simulink model "H16"  (Simulink 7.3)
settings: Solver=ode45  StartTime=0.0  StopTime=2  RelTol=1e-3
undefined symbols (not defined in the file or in its folder): DiscIntNeverNeededParam
libraries: simulink x13
settings Model: Creator=Sainquake  LastModifiedBy=Sainquake

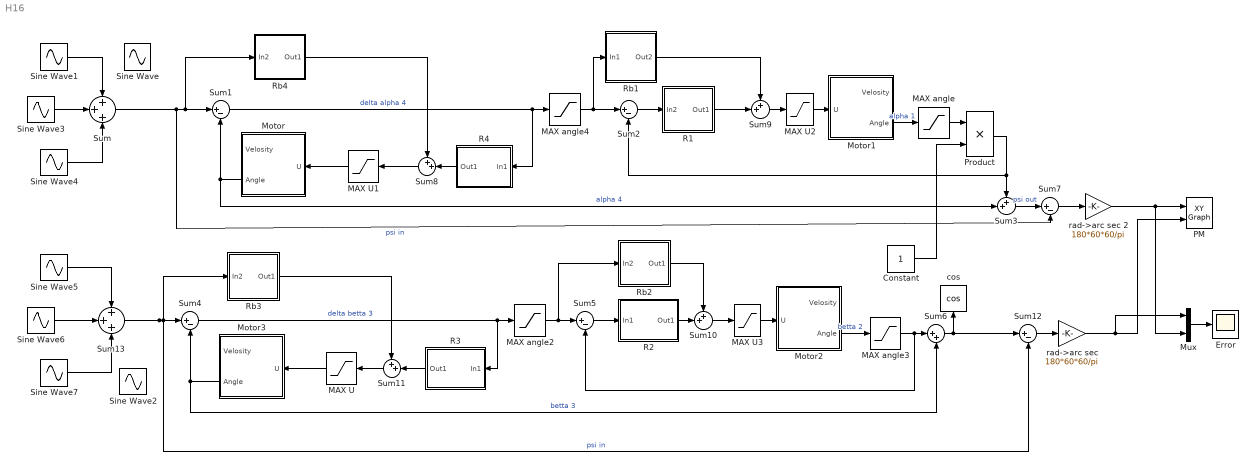
== system H16 ==
  Constant : Constant  OutDataType=fixdt(1, 16)  OutScaling=2^0
  Error : Scope
      settings: YMin=-50  YMax=250  SaveName=ScopeData2  MaxDataPoints=500000
  MAX U : Saturate  UpperLimit=42  LowerLimit=-42
  MAX U1 : Saturate  UpperLimit=42  LowerLimit=-42
  MAX U2 : Saturate  UpperLimit=12  LowerLimit=-12
  MAX U3 : Saturate  UpperLimit=12  LowerLimit=-12
  MAX angle : Saturate  UpperLimit=8/180*3.14  LowerLimit=-8/180*3.14
  MAX angle2 : Saturate  UpperLimit=4/180*3.14  LowerLimit=-4/180*3.14
  MAX angle3 : Saturate  UpperLimit=4/180*3.14  LowerLimit=-4/180*3.14
  MAX angle4 : Saturate  UpperLimit=8/180*3.14  LowerLimit=-8/180*3.14
  Motor : Subsystem  TreatAsAtomicUnit=on
  Motor1 : Subsystem  TreatAsAtomicUnit=on
  Motor2 : Subsystem  TreatAsAtomicUnit=on
  Motor3 : Subsystem  TreatAsAtomicUnit=on
  Mux : Mux  Inputs=2
  PM : simulink/Sinks/XY Graph  SystemSampleTime=-1  xmin=-3*1280  xmax=3*1280  ymin=-3*960  ymax=3*960  st=-1
  Product : Product  OutDataType=fixdt(1, 16)  OutScaling=2^0  RndMeth=Zero
  R1 : Subsystem
  R2 : Subsystem
  R3 : Subsystem
  R4 : Subsystem
  Rb1 : Subsystem
  Rb2 : Subsystem
  Rb3 : Subsystem
  Rb4 : Subsystem
  Sine Wave{,1..2,5} (4 alike) : Sin  Amplitude=1  Bias=0  Frequency=1  Phase=0  Samples=10  SampleTime=0  Offset=0
  Sine Wave3 : Sin  Amplitude=1/10000  Bias=0  Frequency=2*pi*14  Phase=0  Samples=10  SampleTime=0  Offset=0
  Sine Wave4 : Sin  Amplitude=1/400  Bias=0  Frequency=2*pi*4  Phase=0  Samples=10  SampleTime=0  Offset=0
  Sine Wave6 : Sin  Amplitude=1/10000  Bias=0  Frequency=2*pi*14  Phase=0  Samples=10  SampleTime=0  Offset=0
  Sine Wave7 : Sin  Amplitude=1/400  Bias=0  Frequency=2*pi*4  Phase=0  Samples=10  SampleTime=0  Offset=0
  Sum : Sum  Inputs=+++  OutDataType=fixdt(1, 16)  OutScaling=2^0
  Sum{1..2,4..5,7,12} (6 alike) : Sum  Inputs=|+-  OutDataType=fixdt(1, 16)  OutScaling=2^0
  Sum{3,8..11} (5 alike) : Sum  Inputs=++|  OutDataType=fixdt(1, 16)  OutScaling=2^0
  Sum13 : Sum  Inputs=+++  OutDataType=fixdt(1, 16)  OutScaling=2^0
  Sum6 : Sum  Inputs=|++  OutDataType=fixdt(1, 16)  OutScaling=2^0
  cos : Trigonometry  Operator=cos
  rad->arc sec : Gain  Gain=180*60*60/pi  ParameterDataType=fixdt(1, 16)  ParameterScaling=2^0  OutDataType=fixdt(1, 16)  OutScaling=2^0
  rad->arc sec 2 : Gain  Gain=180*60*60/pi  ParameterDataType=fixdt(1, 16)  ParameterScaling=2^0  OutDataType=fixdt(1, 16)  OutScaling=2^0
  wires:
  R4/1(Out1) -> Sum8/2
  Motor1/2(Angle) -> MAX angle/1  "alpha 1"
  Sum2/1 -> R1/1(In2)
  Product/1 -> Sum3/1, Sum2/2
  Sum3/1 -> Sum7/1  "psi out"
  Motor/2(Angle) -> Sum1/2, Sum3/2  "alpha 4"
  R3/1(Out1) -> Sum11/2
  Sum4/1 -> R3/1(In1), MAX angle2/1  "delta betta 3"
  Sum13/1 -> Sum4/1, Rb3/1(In2), Sum12/2  "psi in"
  R2/1(Out1) -> Sum10/2
  Motor2/2(Angle) -> MAX angle3/1  "betta 2"
  Sum5/1 -> R2/1(In1)
  Motor3/2(Angle) -> Sum4/2, Sum6/2  "betta 3"
  Sum6/1 -> cos/1, Sum12/1
  Sum/1 -> Sum1/1, Rb4/1(In2), Sum7/2  "psi in"
  Rb1/1(Out2) -> Sum9/1
  Rb4/1(Out1) -> Sum8/1
  R1/1(Out1) -> Sum9/2
  Sum9/1 -> MAX U2/1
  Rb3/1(Out1) -> Sum11/1
  Sum11/1 -> MAX U/1
  Sum10/1 -> MAX U3/1
  Rb2/1(Out1) -> Sum10/1
  Sum7/1 -> rad->arc sec 2/1
  rad->arc sec 2/1 -> PM/1, Mux/2
  Sum1/1 -> R4/1(In1), MAX angle4/1  "delta alpha 4"
  rad->arc sec/1 -> Mux/1, PM/2
  Sum12/1 -> rad->arc sec/1
  Mux/1 -> Error/1
  MAX angle4/1 -> Sum2/1, Rb1/1(In1)
  MAX angle2/1 -> Sum5/1, Rb2/1(In2)
  MAX U2/1 -> Motor1/1(U)
  MAX U3/1 -> Motor2/1(U)
  MAX angle/1 -> Product/1
  MAX angle3/1 -> Sum5/2, Sum6/1
  Sum8/1 -> MAX U1/1
  MAX U/1 -> Motor3/1(U)
  MAX U1/1 -> Motor/1(U)
  Sine Wave3/1 -> Sum/2
  Sine Wave1/1 -> Sum/1
  Sine Wave6/1 -> Sum13/2
  Sine Wave7/1 -> Sum13/3
  Sine Wave4/1 -> Sum/3
  Sine Wave5/1 -> Sum13/1
  Constant/1 -> Product/2

== system H16/Motor ==
  U : Inport  OutDataType=fixdt(1, 16)  OutScaling=2^0
  Ang : Integrator
  Transfer Fcn3 : TransferFcn  Numerator=[3.87]  Denominator=[16.713 1]
  Velosity : Outport  OutDataType=fixdt(1, 16)  OutScaling=2^0
  Angle : Outport  Port=2  OutDataType=fixdt(1, 16)  OutScaling=2^0
  wires:
  Ang/1 -> Angle/1
  U/1 -> Transfer Fcn3/1
  Transfer Fcn3/1 -> Ang/1, Velosity/1

== system H16/Motor1 ==
  U : Inport  OutDataType=fixdt(1, 16)  OutScaling=2^0
  Ang : Integrator
  Transfer Fcn3 : TransferFcn  Numerator=[8.37]  Denominator=[0.0002343 1]
  Velosity : Outport  OutDataType=fixdt(1, 16)  OutScaling=2^0
  Angle : Outport  Port=2  OutDataType=fixdt(1, 16)  OutScaling=2^0
  wires:
  Ang/1 -> Angle/1
  U/1 -> Transfer Fcn3/1
  Transfer Fcn3/1 -> Ang/1, Velosity/1

== system H16/Motor2 ==
  U : Inport  OutDataType=fixdt(1, 16)  OutScaling=2^0
  Ang : Integrator
  Transfer Fcn3 : TransferFcn  Numerator=[8.37]  Denominator=[0.015 1]
  Velosity : Outport  OutDataType=fixdt(1, 16)  OutScaling=2^0
  Angle : Outport  Port=2  OutDataType=fixdt(1, 16)  OutScaling=2^0
  wires:
  Ang/1 -> Angle/1
  U/1 -> Transfer Fcn3/1
  Transfer Fcn3/1 -> Ang/1, Velosity/1

== system H16/Motor3 ==
  U : Inport  OutDataType=fixdt(1, 16)  OutScaling=2^0
  Ang : Integrator
  Transfer Fcn3 : TransferFcn  Numerator=[3.87]  Denominator=[2.662 1]
  Velosity : Outport  OutDataType=fixdt(1, 16)  OutScaling=2^0
  Angle : Outport  Port=2  OutDataType=fixdt(1, 16)  OutScaling=2^0
  wires:
  Ang/1 -> Angle/1
  U/1 -> Transfer Fcn3/1
  Transfer Fcn3/1 -> Ang/1, Velosity/1

== system H16/R1 ==
  In2 : Inport  OutDataType=fixdt(1, 16)  OutScaling=2^0
  Constan : Constant  Value=1935.48  OutDataType=fixdt(1, 16)  OutScaling=2^0
  Constan1 : Constant  Value=0  OutDataType=fixdt(1, 16)  OutScaling=2^0
  Constan2 : Constant  Value=0.453  OutDataType=fixdt(1, 16)  OutScaling=2^0
  PID : Subsystem
  Out1 : Outport  OutDataType=fixdt(1, 16)  OutScaling=2^0
  wires:
  Constan/1 -> PID/2(p)
  Constan1/1 -> PID/3(i)
  Constan2/1 -> PID/4(d)
  In2/1 -> PID/1(In1)
  PID/1(Out1) -> Out1/1

== system H16/R2 ==
  In1 : Inport  OutDataType=fixdt(1, 16)  OutScaling=2^0
  Constan : Constant  Value=645.161*5  OutDataType=fixdt(1, 16)  OutScaling=2^0
  Constan1 : Constant  Value=0  OutDataType=fixdt(1, 16)  OutScaling=2^0
  Constan2 : Constant  Value=645.161*5*0.015/10  OutDataType=fixdt(1, 16)  OutScaling=2^0
  PID : Subsystem
  Out1 : Outport  OutDataType=fixdt(1, 16)  OutScaling=2^0
  wires:
  Constan/1 -> PID/2(p)
  Constan1/1 -> PID/3(i)
  Constan2/1 -> PID/4(d)
  In1/1 -> PID/1(In1)
  PID/1(Out1) -> Out1/1

== system H16/R3 ==
  In1 : Inport  OutDataType=fixdt(1, 16)  OutScaling=2^0
  Constan : Constant  Value=755/10  OutDataType=fixdt(1, 16)  OutScaling=2^0
  Constan1 : Constant  Value=0  OutDataType=fixdt(1, 16)  OutScaling=2^0
  Constan2 : Constant  Value=2.662*775/10  OutDataType=fixdt(1, 16)  OutScaling=2^0
  PID : Subsystem
  Out1 : Outport  OutDataType=fixdt(1, 16)  OutScaling=2^0
  wires:
  Constan/1 -> PID/2(p)
  Constan1/1 -> PID/3(i)
  Constan2/1 -> PID/4(d)
  In1/1 -> PID/1(In1)
  PID/1(Out1) -> Out1/1

== system H16/R4 ==
  In1 : Inport  OutDataType=fixdt(1, 16)  OutScaling=2^0
  Constan : Constant  Value=755/10  OutDataType=fixdt(1, 16)  OutScaling=2^0
  Constan1 : Constant  Value=0  OutDataType=fixdt(1, 16)  OutScaling=2^0
  Constan2 : Constant  Value=12952.57/10  OutDataType=fixdt(1, 16)  OutScaling=2^0
  PID : Subsystem
  Out1 : Outport  OutDataType=fixdt(1, 16)  OutScaling=2^0
  wires:
  In1/1 -> PID/1(In1)
  Constan/1 -> PID/2(p)
  Constan1/1 -> PID/3(i)
  Constan2/1 -> PID/4(d)
  PID/1(Out1) -> Out1/1

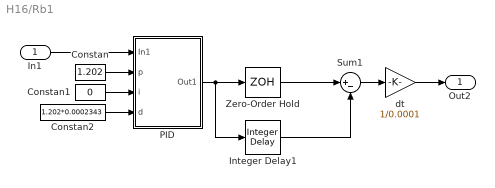
== system H16/Rb1 ==
  In1 : Inport  OutDataType=fixdt(1, 16)  OutScaling=2^0
  Constan : Constant  Value=1.202  OutDataType=fixdt(1, 16)  OutScaling=2^0
  Constan1 : Constant  Value=0  OutDataType=fixdt(1, 16)  OutScaling=2^0
  Constan2 : Constant  Value=1.202*0.0002343  OutDataType=fixdt(1, 16)  OutScaling=2^0
  Integer Delay1 : simulink/Discrete/Integer Delay  vinit=0  samptime=0.0001  NumDelays=1
  PID : Subsystem
  Sum1 : Sum  Inputs=|+-  OutDataType=fixdt(1, 16)  OutScaling=2^0
  Zero-Order Hold : ZeroOrderHold  SampleTime=0.0001
  dt : Gain  Gain=1/0.0001  ParameterDataType=fixdt(1, 16)  ParameterScaling=2^0  OutDataType=fixdt(1, 16)  OutScaling=2^0
  Out2 : Outport  OutDataType=fixdt(1, 16)  OutScaling=2^0
  wires:
  Constan/1 -> PID/2(p)
  Constan1/1 -> PID/3(i)
  Constan2/1 -> PID/4(d)
  Zero-Order Hold/1 -> Sum1/1
  Sum1/1 -> dt/1
  Integer Delay1/1 -> Sum1/2
  PID/1(Out1) -> Integer Delay1/1, Zero-Order Hold/1
  In1/1 -> PID/1(In1)
  dt/1 -> Out2/1

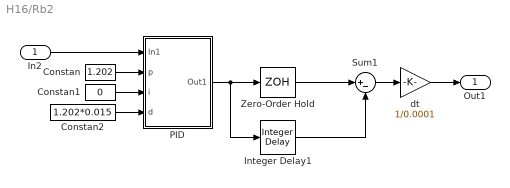
== system H16/Rb2 ==
  In2 : Inport  OutDataType=fixdt(1, 16)  OutScaling=2^0
  Constan : Constant  Value=1.202  OutDataType=fixdt(1, 16)  OutScaling=2^0
  Constan1 : Constant  Value=0  OutDataType=fixdt(1, 16)  OutScaling=2^0
  Constan2 : Constant  Value=1.202*0.015  OutDataType=fixdt(1, 16)  OutScaling=2^0
  Integer Delay1 : simulink/Discrete/Integer Delay  vinit=0  samptime=0.0001  NumDelays=1
  PID : Subsystem
  Sum1 : Sum  Inputs=|+-  OutDataType=fixdt(1, 16)  OutScaling=2^0
  Zero-Order Hold : ZeroOrderHold  SampleTime=0.0001
  dt : Gain  Gain=1/0.0001  ParameterDataType=fixdt(1, 16)  ParameterScaling=2^0  OutDataType=fixdt(1, 16)  OutScaling=2^0
  Out1 : Outport  OutDataType=fixdt(1, 16)  OutScaling=2^0
  wires:
  Constan/1 -> PID/2(p)
  Constan1/1 -> PID/3(i)
  Constan2/1 -> PID/4(d)
  In2/1 -> PID/1(In1)
  Zero-Order Hold/1 -> Sum1/1
  Sum1/1 -> dt/1
  Integer Delay1/1 -> Sum1/2
  PID/1(Out1) -> Integer Delay1/1, Zero-Order Hold/1
  dt/1 -> Out1/1

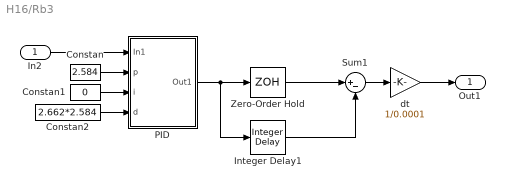
== system H16/Rb3 ==
  In2 : Inport  OutDataType=fixdt(1, 16)  OutScaling=2^0
  Constan : Constant  Value=2.584  OutDataType=fixdt(1, 16)  OutScaling=2^0
  Constan1 : Constant  Value=0  OutDataType=fixdt(1, 16)  OutScaling=2^0
  Constan2 : Constant  Value=2.662*2.584  OutDataType=fixdt(1, 16)  OutScaling=2^0
  Integer Delay1 : simulink/Discrete/Integer Delay  vinit=0  samptime=0.0001  NumDelays=1
  PID : Subsystem
  Sum1 : Sum  Inputs=|+-  OutDataType=fixdt(1, 16)  OutScaling=2^0
  Zero-Order Hold : ZeroOrderHold  SampleTime=0.0001
  dt : Gain  Gain=1/0.0001  ParameterDataType=fixdt(1, 16)  ParameterScaling=2^0  OutDataType=fixdt(1, 16)  OutScaling=2^0
  Out1 : Outport  OutDataType=fixdt(1, 16)  OutScaling=2^0
  wires:
  Constan/1 -> PID/2(p)
  Constan1/1 -> PID/3(i)
  Constan2/1 -> PID/4(d)
  In2/1 -> PID/1(In1)
  Zero-Order Hold/1 -> Sum1/1
  Sum1/1 -> dt/1
  Integer Delay1/1 -> Sum1/2
  PID/1(Out1) -> Integer Delay1/1, Zero-Order Hold/1
  dt/1 -> Out1/1

== system H16/Rb4 ==
  In2 : Inport  OutDataType=fixdt(1, 16)  OutScaling=2^0
  Constan : Constant  Value=2.584  OutDataType=fixdt(1, 16)  OutScaling=2^0
  Constan1 : Constant  Value=0  OutDataType=fixdt(1, 16)  OutScaling=2^0
  Constan2 : Constant  Value=43.1863  OutDataType=fixdt(1, 16)  OutScaling=2^0
  Integer Delay1 : simulink/Discrete/Integer Delay  vinit=0  samptime=0.0001  NumDelays=1
  PID : Subsystem
  Sum1 : Sum  Inputs=|+-  OutDataType=fixdt(1, 16)  OutScaling=2^0
  Zero-Order Hold : ZeroOrderHold  SampleTime=0.0001
  dt : Gain  Gain=1/0.0001  ParameterDataType=fixdt(1, 16)  ParameterScaling=2^0  OutDataType=fixdt(1, 16)  OutScaling=2^0
  Out1 : Outport  OutDataType=fixdt(1, 16)  OutScaling=2^0
  wires:
  Constan/1 -> PID/2(p)
  Constan1/1 -> PID/3(i)
  Constan2/1 -> PID/4(d)
  In2/1 -> PID/1(In1)
  Zero-Order Hold/1 -> Sum1/1
  Sum1/1 -> dt/1
  Integer Delay1/1 -> Sum1/2
  dt/1 -> Out1/1
  PID/1(Out1) -> Zero-Order Hold/1, Integer Delay1/1

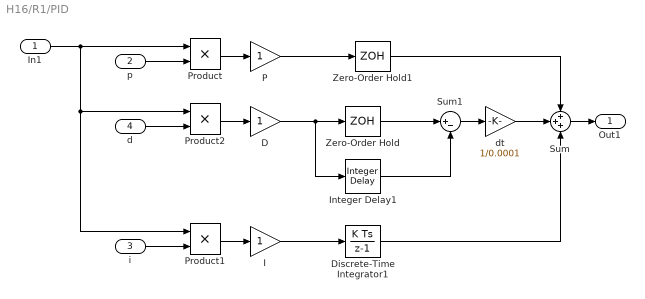
== system H16/R1/PID ==
  In1 : Inport  OutDataType=fixdt(1, 16)  OutScaling=2^0
  p : Inport  Port=2  OutDataType=fixdt(1, 16)  OutScaling=2^0
  i : Inport  Port=3  OutDataType=fixdt(1, 16)  OutScaling=2^0
  d : Inport  Port=4  OutDataType=fixdt(1, 16)  OutScaling=2^0
  D : Gain  ParameterDataType=fixdt(1, 16)  ParameterScaling=2^0  OutDataType=fixdt(1, 16)  OutScaling=2^0
  Discrete-Time Integrator1 : DiscreteIntegrator  SampleTime=0.0001  OutDataType=fixdt(1, 16)  OutScaling=2^0  ICPrevOutput=DiscIntNeverNeededParam  ICPrevScaledInput=DiscIntNeverNeededParam
  I : Gain  ParameterDataType=fixdt(1, 16)  ParameterScaling=2^0  OutDataType=fixdt(1, 16)  OutScaling=2^0
  Integer Delay1 : simulink/Discrete/Integer Delay  vinit=0.0  samptime=0.0001  NumDelays=1
  P : Gain  ParameterDataType=fixdt(1, 16)  ParameterScaling=2^0  OutDataType=fixdt(1, 16)  OutScaling=2^0
  Product : Product  OutDataType=fixdt(1, 16)  OutScaling=2^0  RndMeth=Zero
  Product1 : Product  OutDataType=fixdt(1, 16)  OutScaling=2^0  RndMeth=Zero
  Product2 : Product  OutDataType=fixdt(1, 16)  OutScaling=2^0  RndMeth=Zero
  Sum : Sum  Inputs=+++  OutDataType=fixdt(1, 16)  OutScaling=2^0
  Sum1 : Sum  Inputs=|+-  OutDataType=fixdt(1, 16)  OutScaling=2^0
  Zero-Order Hold : ZeroOrderHold  SampleTime=0.0001
  Zero-Order Hold1 : ZeroOrderHold  SampleTime=0.0001
  dt : Gain  Gain=1/0.0001  ParameterDataType=fixdt(1, 16)  ParameterScaling=2^0  OutDataType=fixdt(1, 16)  OutScaling=2^0
  Out1 : Outport  OutDataType=fixdt(1, 16)  OutScaling=2^0
  wires:
  Zero-Order Hold/1 -> Sum1/1
  Sum1/1 -> dt/1
  Integer Delay1/1 -> Sum1/2
  D/1 -> Integer Delay1/1, Zero-Order Hold/1
  dt/1 -> Sum/2
  Zero-Order Hold1/1 -> Sum/1
  P/1 -> Zero-Order Hold1/1
  I/1 -> Discrete-Time Integrator1/1
  Discrete-Time Integrator1/1 -> Sum/3
  Sum/1 -> Out1/1
  Product/1 -> P/1
  In1/1 -> Product/1, Product2/1, Product1/1
  p/1 -> Product/2
  Product2/1 -> D/1
  Product1/1 -> I/1
  d/1 -> Product2/2
  i/1 -> Product1/2

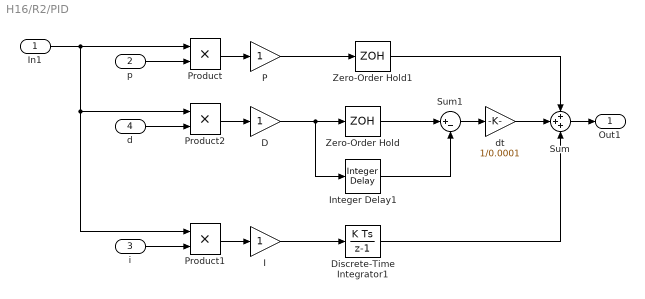
== system H16/R2/PID ==
  In1 : Inport  OutDataType=fixdt(1, 16)  OutScaling=2^0
  p : Inport  Port=2  OutDataType=fixdt(1, 16)  OutScaling=2^0
  i : Inport  Port=3  OutDataType=fixdt(1, 16)  OutScaling=2^0
  d : Inport  Port=4  OutDataType=fixdt(1, 16)  OutScaling=2^0
  D : Gain  ParameterDataType=fixdt(1, 16)  ParameterScaling=2^0  OutDataType=fixdt(1, 16)  OutScaling=2^0
  Discrete-Time Integrator1 : DiscreteIntegrator  SampleTime=0.0001  OutDataType=fixdt(1, 16)  OutScaling=2^0  ICPrevOutput=DiscIntNeverNeededParam  ICPrevScaledInput=DiscIntNeverNeededParam
  I : Gain  ParameterDataType=fixdt(1, 16)  ParameterScaling=2^0  OutDataType=fixdt(1, 16)  OutScaling=2^0
  Integer Delay1 : simulink/Discrete/Integer Delay  vinit=0  samptime=0.0001  NumDelays=1
  P : Gain  ParameterDataType=fixdt(1, 16)  ParameterScaling=2^0  OutDataType=fixdt(1, 16)  OutScaling=2^0
  Product : Product  OutDataType=fixdt(1, 16)  OutScaling=2^0  RndMeth=Zero
  Product1 : Product  OutDataType=fixdt(1, 16)  OutScaling=2^0  RndMeth=Zero
  Product2 : Product  OutDataType=fixdt(1, 16)  OutScaling=2^0  RndMeth=Zero
  Sum : Sum  Inputs=+++  OutDataType=fixdt(1, 16)  OutScaling=2^0
  Sum1 : Sum  Inputs=|+-  OutDataType=fixdt(1, 16)  OutScaling=2^0
  Zero-Order Hold : ZeroOrderHold  SampleTime=0.0001
  Zero-Order Hold1 : ZeroOrderHold  SampleTime=0.0001
  dt : Gain  Gain=1/0.0001  ParameterDataType=fixdt(1, 16)  ParameterScaling=2^0  OutDataType=fixdt(1, 16)  OutScaling=2^0
  Out1 : Outport  OutDataType=fixdt(1, 16)  OutScaling=2^0
  wires:
  Zero-Order Hold/1 -> Sum1/1
  Sum1/1 -> dt/1
  Integer Delay1/1 -> Sum1/2
  D/1 -> Integer Delay1/1, Zero-Order Hold/1
  dt/1 -> Sum/2
  Zero-Order Hold1/1 -> Sum/1
  P/1 -> Zero-Order Hold1/1
  I/1 -> Discrete-Time Integrator1/1
  Discrete-Time Integrator1/1 -> Sum/3
  Sum/1 -> Out1/1
  Product/1 -> P/1
  In1/1 -> Product/1, Product2/1, Product1/1
  p/1 -> Product/2
  Product2/1 -> D/1
  Product1/1 -> I/1
  d/1 -> Product2/2
  i/1 -> Product1/2

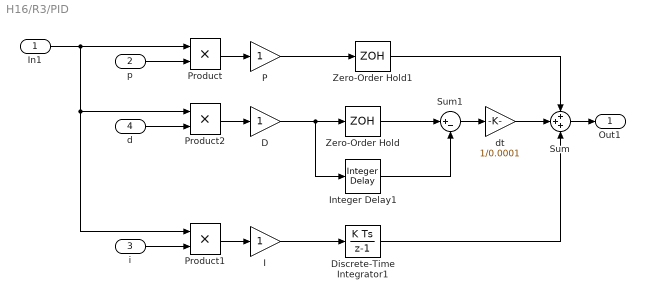
== system H16/R3/PID ==
  In1 : Inport  OutDataType=fixdt(1, 16)  OutScaling=2^0
  p : Inport  Port=2  OutDataType=fixdt(1, 16)  OutScaling=2^0
  i : Inport  Port=3  OutDataType=fixdt(1, 16)  OutScaling=2^0
  d : Inport  Port=4  OutDataType=fixdt(1, 16)  OutScaling=2^0
  D : Gain  ParameterDataType=fixdt(1, 16)  ParameterScaling=2^0  OutDataType=fixdt(1, 16)  OutScaling=2^0
  Discrete-Time Integrator1 : DiscreteIntegrator  SampleTime=0.0001  OutDataType=fixdt(1, 16)  OutScaling=2^0  ICPrevOutput=DiscIntNeverNeededParam  ICPrevScaledInput=DiscIntNeverNeededParam
  I : Gain  ParameterDataType=fixdt(1, 16)  ParameterScaling=2^0  OutDataType=fixdt(1, 16)  OutScaling=2^0
  Integer Delay1 : simulink/Discrete/Integer Delay  vinit=0  samptime=0.0001  NumDelays=1
  P : Gain  ParameterDataType=fixdt(1, 16)  ParameterScaling=2^0  OutDataType=fixdt(1, 16)  OutScaling=2^0
  Product : Product  OutDataType=fixdt(1, 16)  OutScaling=2^0  RndMeth=Zero
  Product1 : Product  OutDataType=fixdt(1, 16)  OutScaling=2^0  RndMeth=Zero
  Product2 : Product  OutDataType=fixdt(1, 16)  OutScaling=2^0  RndMeth=Zero
  Sum : Sum  Inputs=+++  OutDataType=fixdt(1, 16)  OutScaling=2^0
  Sum1 : Sum  Inputs=|+-  OutDataType=fixdt(1, 16)  OutScaling=2^0
  Zero-Order Hold : ZeroOrderHold  SampleTime=0.0001
  Zero-Order Hold1 : ZeroOrderHold  SampleTime=0.0001
  dt : Gain  Gain=1/0.0001  ParameterDataType=fixdt(1, 16)  ParameterScaling=2^0  OutDataType=fixdt(1, 16)  OutScaling=2^0
  Out1 : Outport  OutDataType=fixdt(1, 16)  OutScaling=2^0
  wires:
  Zero-Order Hold/1 -> Sum1/1
  Sum1/1 -> dt/1
  Integer Delay1/1 -> Sum1/2
  D/1 -> Integer Delay1/1, Zero-Order Hold/1
  dt/1 -> Sum/2
  Zero-Order Hold1/1 -> Sum/1
  P/1 -> Zero-Order Hold1/1
  I/1 -> Discrete-Time Integrator1/1
  Discrete-Time Integrator1/1 -> Sum/3
  Sum/1 -> Out1/1
  Product/1 -> P/1
  In1/1 -> Product/1, Product2/1, Product1/1
  p/1 -> Product/2
  Product2/1 -> D/1
  Product1/1 -> I/1
  d/1 -> Product2/2
  i/1 -> Product1/2

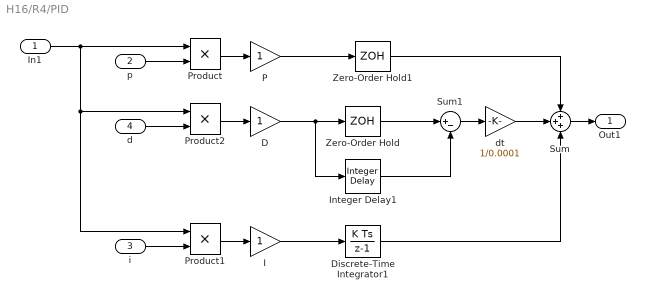
== system H16/R4/PID ==
  In1 : Inport  OutDataType=fixdt(1, 16)  OutScaling=2^0
  p : Inport  Port=2  OutDataType=fixdt(1, 16)  OutScaling=2^0
  i : Inport  Port=3  OutDataType=fixdt(1, 16)  OutScaling=2^0
  d : Inport  Port=4  OutDataType=fixdt(1, 16)  OutScaling=2^0
  D : Gain  ParameterDataType=fixdt(1, 16)  ParameterScaling=2^0  OutDataType=fixdt(1, 16)  OutScaling=2^0
  Discrete-Time Integrator1 : DiscreteIntegrator  SampleTime=0.0001  OutDataType=fixdt(1, 16)  OutScaling=2^0  ICPrevOutput=DiscIntNeverNeededParam  ICPrevScaledInput=DiscIntNeverNeededParam
  I : Gain  ParameterDataType=fixdt(1, 16)  ParameterScaling=2^0  OutDataType=fixdt(1, 16)  OutScaling=2^0
  Integer Delay1 : simulink/Discrete/Integer Delay  vinit=0  samptime=0.0001  NumDelays=1
  P : Gain  ParameterDataType=fixdt(1, 16)  ParameterScaling=2^0  OutDataType=fixdt(1, 16)  OutScaling=2^0
  Product : Product  OutDataType=fixdt(1, 16)  OutScaling=2^0  RndMeth=Zero
  Product1 : Product  OutDataType=fixdt(1, 16)  OutScaling=2^0  RndMeth=Zero
  Product2 : Product  OutDataType=fixdt(1, 16)  OutScaling=2^0  RndMeth=Zero
  Sum : Sum  Inputs=+++  OutDataType=fixdt(1, 16)  OutScaling=2^0
  Sum1 : Sum  Inputs=|+-  OutDataType=fixdt(1, 16)  OutScaling=2^0
  Zero-Order Hold : ZeroOrderHold  SampleTime=0.0001
  Zero-Order Hold1 : ZeroOrderHold  SampleTime=0.0001
  dt : Gain  Gain=1/0.0001  ParameterDataType=fixdt(1, 16)  ParameterScaling=2^0  OutDataType=fixdt(1, 16)  OutScaling=2^0
  Out1 : Outport  OutDataType=fixdt(1, 16)  OutScaling=2^0
  wires:
  Zero-Order Hold/1 -> Sum1/1
  Sum1/1 -> dt/1
  Integer Delay1/1 -> Sum1/2
  D/1 -> Integer Delay1/1, Zero-Order Hold/1
  dt/1 -> Sum/2
  Zero-Order Hold1/1 -> Sum/1
  P/1 -> Zero-Order Hold1/1
  I/1 -> Discrete-Time Integrator1/1
  Discrete-Time Integrator1/1 -> Sum/3
  Sum/1 -> Out1/1
  Product/1 -> P/1
  In1/1 -> Product/1, Product2/1, Product1/1
  p/1 -> Product/2
  Product2/1 -> D/1
  Product1/1 -> I/1
  d/1 -> Product2/2
  i/1 -> Product1/2

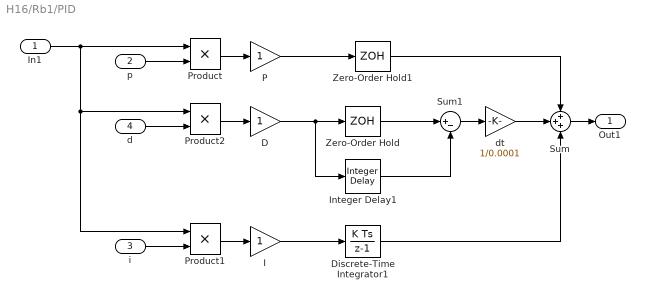
== system H16/Rb1/PID ==
  In1 : Inport  OutDataType=fixdt(1, 16)  OutScaling=2^0
  p : Inport  Port=2  OutDataType=fixdt(1, 16)  OutScaling=2^0
  i : Inport  Port=3  OutDataType=fixdt(1, 16)  OutScaling=2^0
  d : Inport  Port=4  OutDataType=fixdt(1, 16)  OutScaling=2^0
  D : Gain  ParameterDataType=fixdt(1, 16)  ParameterScaling=2^0  OutDataType=fixdt(1, 16)  OutScaling=2^0
  Discrete-Time Integrator1 : DiscreteIntegrator  SampleTime=0.0001  OutDataType=fixdt(1, 16)  OutScaling=2^0  ICPrevOutput=DiscIntNeverNeededParam  ICPrevScaledInput=DiscIntNeverNeededParam
  I : Gain  ParameterDataType=fixdt(1, 16)  ParameterScaling=2^0  OutDataType=fixdt(1, 16)  OutScaling=2^0
  Integer Delay1 : simulink/Discrete/Integer Delay  vinit=0  samptime=0.0001  NumDelays=1
  P : Gain  ParameterDataType=fixdt(1, 16)  ParameterScaling=2^0  OutDataType=fixdt(1, 16)  OutScaling=2^0
  Product : Product  OutDataType=fixdt(1, 16)  OutScaling=2^0  RndMeth=Zero
  Product1 : Product  OutDataType=fixdt(1, 16)  OutScaling=2^0  RndMeth=Zero
  Product2 : Product  OutDataType=fixdt(1, 16)  OutScaling=2^0  RndMeth=Zero
  Sum : Sum  Inputs=+++  OutDataType=fixdt(1, 16)  OutScaling=2^0
  Sum1 : Sum  Inputs=|+-  OutDataType=fixdt(1, 16)  OutScaling=2^0
  Zero-Order Hold : ZeroOrderHold  SampleTime=0.0001
  Zero-Order Hold1 : ZeroOrderHold  SampleTime=0.0001
  dt : Gain  Gain=1/0.0001  ParameterDataType=fixdt(1, 16)  ParameterScaling=2^0  OutDataType=fixdt(1, 16)  OutScaling=2^0
  Out1 : Outport  OutDataType=fixdt(1, 16)  OutScaling=2^0
  wires:
  Zero-Order Hold/1 -> Sum1/1
  Sum1/1 -> dt/1
  Integer Delay1/1 -> Sum1/2
  D/1 -> Integer Delay1/1, Zero-Order Hold/1
  dt/1 -> Sum/2
  Zero-Order Hold1/1 -> Sum/1
  P/1 -> Zero-Order Hold1/1
  I/1 -> Discrete-Time Integrator1/1
  Discrete-Time Integrator1/1 -> Sum/3
  Sum/1 -> Out1/1
  Product/1 -> P/1
  In1/1 -> Product/1, Product2/1, Product1/1
  p/1 -> Product/2
  Product2/1 -> D/1
  Product1/1 -> I/1
  d/1 -> Product2/2
  i/1 -> Product1/2

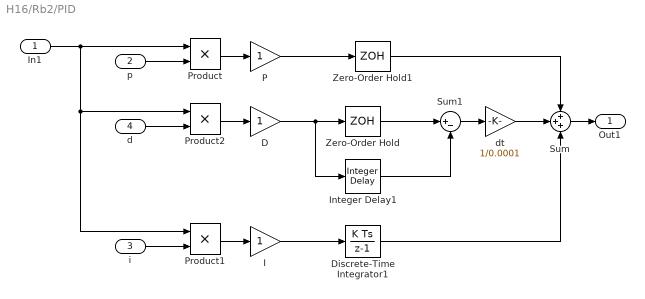
== system H16/Rb2/PID ==
  In1 : Inport  OutDataType=fixdt(1, 16)  OutScaling=2^0
  p : Inport  Port=2  OutDataType=fixdt(1, 16)  OutScaling=2^0
  i : Inport  Port=3  OutDataType=fixdt(1, 16)  OutScaling=2^0
  d : Inport  Port=4  OutDataType=fixdt(1, 16)  OutScaling=2^0
  D : Gain  ParameterDataType=fixdt(1, 16)  ParameterScaling=2^0  OutDataType=fixdt(1, 16)  OutScaling=2^0
  Discrete-Time Integrator1 : DiscreteIntegrator  SampleTime=0.0001  OutDataType=fixdt(1, 16)  OutScaling=2^0  ICPrevOutput=DiscIntNeverNeededParam  ICPrevScaledInput=DiscIntNeverNeededParam
  I : Gain  ParameterDataType=fixdt(1, 16)  ParameterScaling=2^0  OutDataType=fixdt(1, 16)  OutScaling=2^0
  Integer Delay1 : simulink/Discrete/Integer Delay  vinit=0  samptime=0.0001  NumDelays=1
  P : Gain  ParameterDataType=fixdt(1, 16)  ParameterScaling=2^0  OutDataType=fixdt(1, 16)  OutScaling=2^0
  Product : Product  OutDataType=fixdt(1, 16)  OutScaling=2^0  RndMeth=Zero
  Product1 : Product  OutDataType=fixdt(1, 16)  OutScaling=2^0  RndMeth=Zero
  Product2 : Product  OutDataType=fixdt(1, 16)  OutScaling=2^0  RndMeth=Zero
  Sum : Sum  Inputs=+++  OutDataType=fixdt(1, 16)  OutScaling=2^0
  Sum1 : Sum  Inputs=|+-  OutDataType=fixdt(1, 16)  OutScaling=2^0
  Zero-Order Hold : ZeroOrderHold  SampleTime=0.0001
  Zero-Order Hold1 : ZeroOrderHold  SampleTime=0.0001
  dt : Gain  Gain=1/0.0001  ParameterDataType=fixdt(1, 16)  ParameterScaling=2^0  OutDataType=fixdt(1, 16)  OutScaling=2^0
  Out1 : Outport  OutDataType=fixdt(1, 16)  OutScaling=2^0
  wires:
  Zero-Order Hold/1 -> Sum1/1
  Sum1/1 -> dt/1
  Integer Delay1/1 -> Sum1/2
  D/1 -> Integer Delay1/1, Zero-Order Hold/1
  dt/1 -> Sum/2
  Zero-Order Hold1/1 -> Sum/1
  P/1 -> Zero-Order Hold1/1
  I/1 -> Discrete-Time Integrator1/1
  Discrete-Time Integrator1/1 -> Sum/3
  Sum/1 -> Out1/1
  Product/1 -> P/1
  In1/1 -> Product/1, Product2/1, Product1/1
  p/1 -> Product/2
  Product2/1 -> D/1
  Product1/1 -> I/1
  d/1 -> Product2/2
  i/1 -> Product1/2

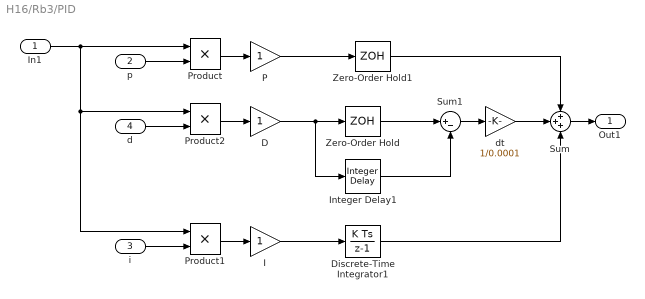
== system H16/Rb3/PID ==
  In1 : Inport  OutDataType=fixdt(1, 16)  OutScaling=2^0
  p : Inport  Port=2  OutDataType=fixdt(1, 16)  OutScaling=2^0
  i : Inport  Port=3  OutDataType=fixdt(1, 16)  OutScaling=2^0
  d : Inport  Port=4  OutDataType=fixdt(1, 16)  OutScaling=2^0
  D : Gain  ParameterDataType=fixdt(1, 16)  ParameterScaling=2^0  OutDataType=fixdt(1, 16)  OutScaling=2^0
  Discrete-Time Integrator1 : DiscreteIntegrator  SampleTime=0.0001  OutDataType=fixdt(1, 16)  OutScaling=2^0  ICPrevOutput=DiscIntNeverNeededParam  ICPrevScaledInput=DiscIntNeverNeededParam
  I : Gain  ParameterDataType=fixdt(1, 16)  ParameterScaling=2^0  OutDataType=fixdt(1, 16)  OutScaling=2^0
  Integer Delay1 : simulink/Discrete/Integer Delay  vinit=0  samptime=0.0001  NumDelays=1
  P : Gain  ParameterDataType=fixdt(1, 16)  ParameterScaling=2^0  OutDataType=fixdt(1, 16)  OutScaling=2^0
  Product : Product  OutDataType=fixdt(1, 16)  OutScaling=2^0  RndMeth=Zero
  Product1 : Product  OutDataType=fixdt(1, 16)  OutScaling=2^0  RndMeth=Zero
  Product2 : Product  OutDataType=fixdt(1, 16)  OutScaling=2^0  RndMeth=Zero
  Sum : Sum  Inputs=+++  OutDataType=fixdt(1, 16)  OutScaling=2^0
  Sum1 : Sum  Inputs=|+-  OutDataType=fixdt(1, 16)  OutScaling=2^0
  Zero-Order Hold : ZeroOrderHold  SampleTime=0.0001
  Zero-Order Hold1 : ZeroOrderHold  SampleTime=0.0001
  dt : Gain  Gain=1/0.0001  ParameterDataType=fixdt(1, 16)  ParameterScaling=2^0  OutDataType=fixdt(1, 16)  OutScaling=2^0
  Out1 : Outport  OutDataType=fixdt(1, 16)  OutScaling=2^0
  wires:
  Zero-Order Hold/1 -> Sum1/1
  Sum1/1 -> dt/1
  Integer Delay1/1 -> Sum1/2
  D/1 -> Integer Delay1/1, Zero-Order Hold/1
  dt/1 -> Sum/2
  Zero-Order Hold1/1 -> Sum/1
  P/1 -> Zero-Order Hold1/1
  I/1 -> Discrete-Time Integrator1/1
  Discrete-Time Integrator1/1 -> Sum/3
  Sum/1 -> Out1/1
  Product/1 -> P/1
  In1/1 -> Product/1, Product2/1, Product1/1
  p/1 -> Product/2
  Product2/1 -> D/1
  Product1/1 -> I/1
  d/1 -> Product2/2
  i/1 -> Product1/2

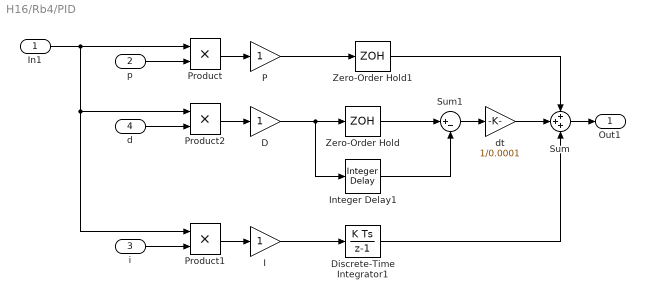
== system H16/Rb4/PID ==
  In1 : Inport  OutDataType=fixdt(1, 16)  OutScaling=2^0
  p : Inport  Port=2  OutDataType=fixdt(1, 16)  OutScaling=2^0
  i : Inport  Port=3  OutDataType=fixdt(1, 16)  OutScaling=2^0
  d : Inport  Port=4  OutDataType=fixdt(1, 16)  OutScaling=2^0
  D : Gain  ParameterDataType=fixdt(1, 16)  ParameterScaling=2^0  OutDataType=fixdt(1, 16)  OutScaling=2^0
  Discrete-Time Integrator1 : DiscreteIntegrator  SampleTime=0.0001  OutDataType=fixdt(1, 16)  OutScaling=2^0  ICPrevOutput=DiscIntNeverNeededParam  ICPrevScaledInput=DiscIntNeverNeededParam
  I : Gain  ParameterDataType=fixdt(1, 16)  ParameterScaling=2^0  OutDataType=fixdt(1, 16)  OutScaling=2^0
  Integer Delay1 : simulink/Discrete/Integer Delay  vinit=0  samptime=0.0001  NumDelays=1
  P : Gain  ParameterDataType=fixdt(1, 16)  ParameterScaling=2^0  OutDataType=fixdt(1, 16)  OutScaling=2^0
  Product : Product  OutDataType=fixdt(1, 16)  OutScaling=2^0  RndMeth=Zero
  Product1 : Product  OutDataType=fixdt(1, 16)  OutScaling=2^0  RndMeth=Zero
  Product2 : Product  OutDataType=fixdt(1, 16)  OutScaling=2^0  RndMeth=Zero
  Sum : Sum  Inputs=+++  OutDataType=fixdt(1, 16)  OutScaling=2^0
  Sum1 : Sum  Inputs=|+-  OutDataType=fixdt(1, 16)  OutScaling=2^0
  Zero-Order Hold : ZeroOrderHold  SampleTime=0.0001
  Zero-Order Hold1 : ZeroOrderHold  SampleTime=0.0001
  dt : Gain  Gain=1/0.0001  ParameterDataType=fixdt(1, 16)  ParameterScaling=2^0  OutDataType=fixdt(1, 16)  OutScaling=2^0
  Out1 : Outport  OutDataType=fixdt(1, 16)  OutScaling=2^0
  wires:
  Zero-Order Hold/1 -> Sum1/1
  Sum1/1 -> dt/1
  Integer Delay1/1 -> Sum1/2
  D/1 -> Integer Delay1/1, Zero-Order Hold/1
  dt/1 -> Sum/2
  Zero-Order Hold1/1 -> Sum/1
  P/1 -> Zero-Order Hold1/1
  I/1 -> Discrete-Time Integrator1/1
  Discrete-Time Integrator1/1 -> Sum/3
  Sum/1 -> Out1/1
  Product/1 -> P/1
  In1/1 -> Product/1, Product2/1, Product1/1
  p/1 -> Product/2
  Product2/1 -> D/1
  Product1/1 -> I/1
  d/1 -> Product2/2
  i/1 -> Product1/2
